simulink model "SMIB_pss"  (Simulink 8.7)
settings: Solver=ode3  StartTime=0.0  StopTime=10  FixedStep=1e-2  MaxStep=1e-2  RelTol=1e-5
values from neighbouring files (symbols this model uses):
  D = 0.0    (= 0)    [initDyn.m]
  delta0 = angle(v(2)+(Rs+1j*Xq)*IG0)    [initDyn.m]
  Efd0 = Epq0+(Xd-Xpd)*Id0    [initDyn.m]
  Epd0 = (Xq-Xpq)*Iq0    [initDyn.m]
  Epq0 = Vq0+Rs*Iq0+Xpd*Id0    [initDyn.m]
  event = [0 1 1.1 10 ... (first row only)    [initDyn.m]
  faulut_3ph = [ ... (first row only)    [initDyn.m]
  fYred = Yred    [initDyn.m]
  KA = ExData(:,1)    [initDyn.m]
  Kpss = KG*T1*T3/(T2*T4)    [initSSA.m]    (also in pss_test.m)
  M = 2*H/ws    [initDyn.m]
  small_d = [ ... (first row only)    [initDyn.m]
  T1 = x(2)    [initSSA.m]    (also in pss_test.m)
  T2 = x(3)    [initSSA.m]    (also in pss_test.m)
  T3 = x(4)    [initSSA.m]    (also in pss_test.m)
  T4 = x(5)    [initSSA.m]    (also in pss_test.m)
  TA = ExData(:,2)    [initDyn.m]
  Tpd0 = GenData(:,6)    [initDyn.m]
  Tpq0 = GenData(:,7)    [initDyn.m]
  Tw = 10    [initSSA.m]    (also in pss_test.m)
  Vinf = V0(1)    [initDyn.m]
  Vref1 = V0(2)+Efd0/KA    [initDyn.m]
  ws = 377    [initDyn.m]
  XXdpd = [Xd-Xpd]    [initDyn.m]
  XXpdq = [Xpq-Xpd]    [initDyn.m]
  XXqpq = [Xq-Xpq]    [initDyn.m]
  Yred = YN    [initDyn.m]
  Zdq = [Rsm -Xpqm;Xpdm Rsm]    [initDyn.m]
libraries: powerlib_extras x3
settings Model: Creator=hbeiran  LastModifiedBy=EBUKA
settings SolverCC: AlgebraicLoopSolver=LineSearch
settings DataIOCC: LimitDataPoints=off  SignalLoggingSaveFormat=ModelDataLogs
settings OptimizationCC: ExpressionDepthLimit=2147483647
settings DebuggingCC: AlgebraicLoopMsg=none  SolverPrmCheckMsg=warning  FcnCallInpInsideContextMsg=UseLocalSettings  StateNameClashWarn=warning
settings SFSimCC: SimParseCustomCode=off
settings GRTTargetCC: CombineOutputUpdateFcns=off  GRTInterface=on

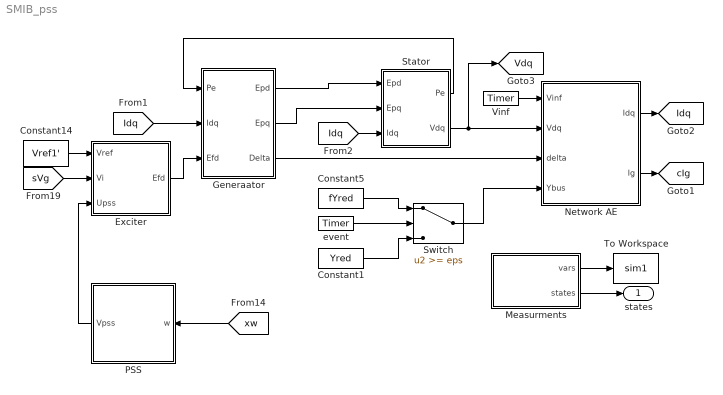
== system SMIB_pss ==
  Constant1 : Constant  Value=Yred  VectorParams1D=off
  Constant14 : Constant  Value=Vref1'  VectorParams1D=off
  Constant5 : Constant  Value=fYred  VectorParams1D=off
  Exciter : Subsystem
  Generaator : Subsystem
  Measurments : Subsystem
  Network AE : MATLAB Function  TreatAsAtomicUnit=on
  PSS : Subsystem
  Stator : Subsystem
  Switch : Switch  Threshold=eps
  To Workspace : ToWorkspace  VariableName=sim1  SaveFormat=Structure With Time  SampleTime=-1
  Vinf : powerlib_extras/Control  Blocks/Timer  t=faulut_3ph(1,:)  e=faulut_3ph(2,:)*Vinf
  event : powerlib_extras/Control  Blocks/Timer  t=event(1,:)  e=event(2,:)
  states : Outport
  tag scope: Idq=global, Vdq=global, cIg=global
  wires:
  Exciter/1(Efd) -> Generaator/3(Efd)
  Constant14/1 -> Exciter/1(Vref)
  [Idq] -> Generaator/2(Idq)
  Network AE/1(Idq) -> [Idq]
  event/1 -> Switch/2
  Constant5/1 -> Switch/1
  Constant1/1 -> Switch/3
  Switch/1 -> Network AE/4(Ybus)
  Measurments/1(vars) -> To Workspace/1
  Measurments/2(states) -> states/1
  Network AE/2(Ig) -> [cIg]
  Stator/2(Vdq) -> [Vdq], Network AE/2(Vdq)
  [Idq] -> Stator/3(Idq)
  Generaator/1(Epd) -> Stator/1(Epd)
  Generaator/2(Epq) -> Stator/2(Epq)
  Stator/1(Pe) -> Generaator/1(Pe)
  [sVg] -> Exciter/2(Vi)
  Vinf/1 -> Network AE/1(Vinf)
  Generaator/3(Delta) -> Network AE/3(delta)
  [xw] -> PSS/1(w)
  PSS/1(Vpss) -> Exciter/3(Upss)

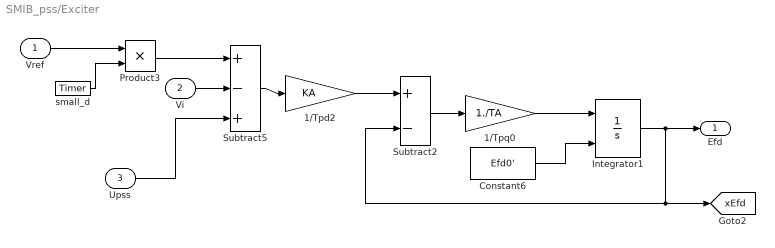
== system SMIB_pss/Exciter ==
  Vref : Inport
  Vi : Inport  Port=2
  Upss : Inport  Port=3
  1/Tpd2 : Gain  Gain=KA
  1/Tpq0 : Gain  Gain=1./TA
  Constant6 : Constant  Value=Efd0'  VectorParams1D=off
  Integrator1 : Integrator  InitialConditionSource=external
  Product3 : Product  RndMeth=Zero
  Subtract2 : Sum  Inputs=+-
  Subtract5 : Sum  Inputs=+-+
  small_d : powerlib_extras/Control  Blocks/Timer  t=small_d(1,:)  e=small_d(2,:)
  Efd : Outport
  tag scope: xEfd=global
  wires:
  Constant6/1 -> Integrator1/2
  Subtract2/1 -> 1/Tpq0/1
  1/Tpq0/1 -> Integrator1/1
  Integrator1/1 -> Efd/1, Subtract2/2, [xEfd]
  Vi/1 -> Subtract5/2
  Subtract5/1 -> 1/Tpd2/1
  1/Tpd2/1 -> Subtract2/1
  small_d/1 -> Product3/2
  Product3/1 -> Subtract5/1
  Vref/1 -> Product3/1
  Upss/1 -> Subtract5/3

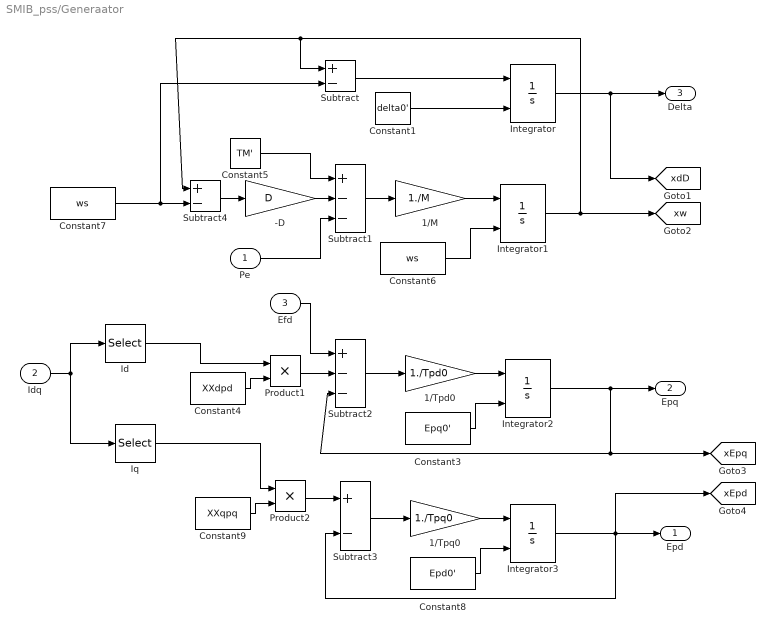
== system SMIB_pss/Generaator ==
  Pe : Inport
  Idq : Inport  Port=2
  Efd : Inport  Port=3
  -D : Gain  Gain=D
  1/M : Gain  Gain=1./M
  1/Tpd0 : Gain  Gain=1./Tpd0
  1/Tpq0 : Gain  Gain=1./Tpq0
  Constant1 : Constant  Value=delta0'  VectorParams1D=off
  Constant3 : Constant  Value=Epq0'  VectorParams1D=off
  Constant4 : Constant  Value=XXdpd  VectorParams1D=off
  Constant5 : Constant  Value=TM'  VectorParams1D=off
  Constant6 : Constant  Value=ws  VectorParams1D=off
  Constant7 : Constant  Value=ws  VectorParams1D=off
  Constant8 : Constant  Value=Epd0'  VectorParams1D=off
  Constant9 : Constant  Value=XXqpq  VectorParams1D=off
  Id : Selector  InputPortWidth=2  IndexOptions=Index vector (dialog)  Indices=[1]  OutputSizes=1
  Integrator{,1..3} (4 alike) : Integrator  InitialConditionSource=external
  Iq : Selector  InputPortWidth=2  IndexOptions=Index vector (dialog)  Indices=[2]  OutputSizes=1
  Product1 : Product  RndMeth=Zero
  Product2 : Product  RndMeth=Zero
  Subtract : Sum  Inputs=+-
  Subtract1 : Sum  Inputs=+--
  Subtract2 : Sum  Inputs=+--
  Subtract3 : Sum  Inputs=+-
  Subtract4 : Sum  Inputs=+-
  Epd : Outport
  Epq : Outport  Port=2
  Delta : Outport  Port=3
  tag scope: xEpd=global, xEpq=global, xdD=global, xw=global
  wires:
  Subtract/1 -> Integrator/1
  Constant5/1 -> Subtract1/1
  Subtract1/1 -> 1/M/1
  1/M/1 -> Integrator1/1
  Constant6/1 -> Integrator1/2
  -D/1 -> Subtract1/2
  Constant3/1 -> Integrator2/2
  Subtract2/1 -> 1/Tpd0/1
  Integrator2/1 -> Epq/1, Subtract2/3, [xEpq]
  Product1/1 -> Subtract2/2
  Constant4/1 -> Product1/2
  1/Tpd0/1 -> Integrator2/1
  Constant8/1 -> Integrator3/2
  Subtract3/1 -> 1/Tpq0/1
  Integrator3/1 -> Epd/1, [xEpd], Subtract3/2
  Constant9/1 -> Product2/2
  1/Tpq0/1 -> Integrator3/1
  Product2/1 -> Subtract3/1
  Efd/1 -> Subtract2/1
  Integrator1/1 -> Subtract/1, Subtract4/1, [xw]
  Id/1 -> Product1/1
  Idq/1 -> Id/1, Iq/1
  Iq/1 -> Product2/1
  Pe/1 -> Subtract1/3
  Integrator/1 -> Delta/1, [xdD]
  Subtract4/1 -> -D/1
  Constant7/1 -> Subtract4/2, Subtract/2
  Constant1/1 -> Integrator/2

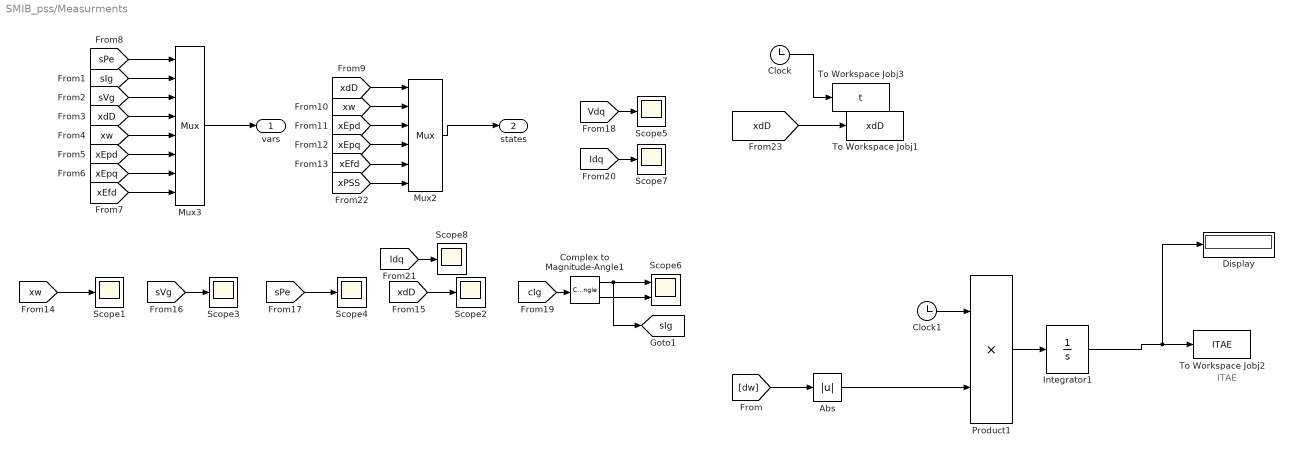
== system SMIB_pss/Measurments ==
  note: ITAE
  Abs : Abs
  Clock : Clock
  Clock1 : Clock
  Complex to Magnitude-Angle1 : ComplexToMagnitudeAngle
  Display : Display
  Integrator1 : Integrator
  Mux2 : Mux  Inputs=6
  Mux3 : Mux  Inputs=8
  Product1 : Product
  Scope{1..5,7..8} (7 alike) : Scope
  Scope6 : Scope  NumInputPorts=2
  To Workspace Jobj1 : ToWorkspace  VariableName=xdD  SampleTime=-1
  To Workspace Jobj2 : ToWorkspace  VariableName=ITAE  SampleTime=-1
  To Workspace Jobj3 : ToWorkspace  VariableName=t  SampleTime=-1
  vars : Outport
  states : Outport  Port=2
  tag scope: sIg=global
  wires:
  Mux3/1 -> vars/1
  [sPe] -> Mux3/1
  [sIg] -> Mux3/2
  [sVg] -> Mux3/3
  [xdD] -> Mux3/4
  [xw] -> Mux3/5
  [xEpd] -> Mux3/6
  [xEpq] -> Mux3/7
  [xEfd] -> Mux3/8
  [xw] -> Mux2/2
  [xEpd] -> Mux2/3
  [xEpq] -> Mux2/4
  [xEfd] -> Mux2/5
  [xdD] -> Mux2/1
  Mux2/1 -> states/1
  [xw] -> Scope1/1
  [xdD] -> Scope2/1
  [sVg] -> Scope3/1
  [sPe] -> Scope4/1
  Complex to Magnitude-Angle1/1 -> Scope6/1, [sIg]
  Complex to Magnitude-Angle1/2 -> Scope6/2
  [cIg] -> Complex to Magnitude-Angle1/1
  [Vdq] -> Scope5/1
  [Idq] -> Scope7/1
  [Idq] -> Scope8/1
  [xPSS] -> Mux2/6
  Clock/1 -> To Workspace Jobj3/1
  [xdD] -> To Workspace Jobj1/1
  Abs/1 -> Product1/2
  [dw] -> Abs/1
  Integrator1/1 -> Display/1, To Workspace Jobj2/1
  Clock1/1 -> Product1/1
  Product1/1 -> Integrator1/1

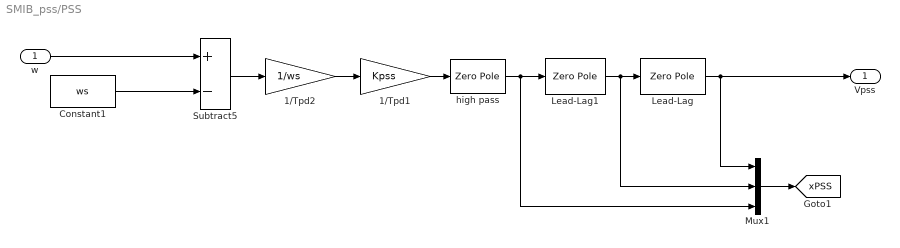
== system SMIB_pss/PSS ==
  w : Inport
  1/Tpd1 : Gain  Gain=Kpss
  1/Tpd2 : Gain  Gain=1/ws
  Constant1 : Constant  Value=ws  VectorParams1D=off
  Lead-Lag : ZeroPole  Zeros=[-1/T3]  Poles=[-1/T4]
  Lead-Lag1 : ZeroPole  Zeros=[-1/T1]  Poles=[-1/T2]
  Mux1 : Mux  Inputs=3
  Subtract5 : Sum  Inputs=+-
  high pass : ZeroPole  Zeros=[0]  Poles=[-1/Tw]
  Vpss : Outport
  tag scope: xPSS=global
  wires:
  Subtract5/1 -> 1/Tpd2/1
  1/Tpd1/1 -> high pass/1
  high pass/1 -> Lead-Lag1/1, Mux1/3
  Lead-Lag1/1 -> Lead-Lag/1, Mux1/2
  Mux1/1 -> [xPSS]
  1/Tpd2/1 -> 1/Tpd1/1
  Lead-Lag/1 -> Vpss/1, Mux1/1
  w/1 -> Subtract5/1
  Constant1/1 -> Subtract5/2

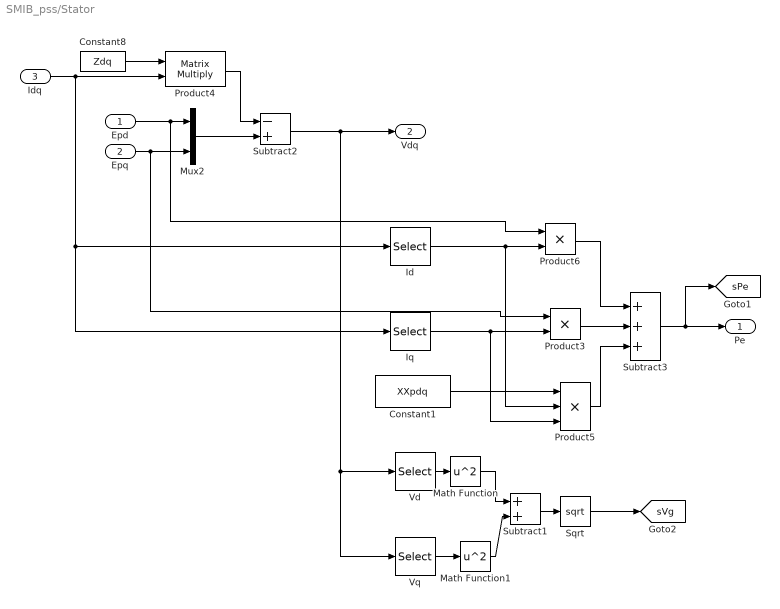
== system SMIB_pss/Stator ==
  Epd : Inport
  Epq : Inport  Port=2
  Idq : Inport  Port=3
  Constant1 : Constant  Value=XXpdq  VectorParams1D=off
  Constant8 : Constant  Value=Zdq  VectorParams1D=off
  Id : Selector  InputPortWidth=2  IndexOptions=Index vector (dialog)  Indices=[1]  OutputSizes=1
  Iq : Selector  InputPortWidth=2  IndexOptions=Index vector (dialog)  Indices=[2]  OutputSizes=1
  Math Function : Math  Operator=square  SaturateOnIntegerOverflow=on
  Math Function1 : Math  Operator=square  SaturateOnIntegerOverflow=on
  Mux2 : Mux  Inputs=2
  Product3 : Product  RndMeth=Zero
  Product4 : Product  Multiplication=Matrix(*)  RndMeth=Zero
  Product5 : Product  Inputs=3  RndMeth=Zero
  Product6 : Product  RndMeth=Zero
  Sqrt : Sqrt  SaturateOnIntegerOverflow=on
  Subtract1 : Sum
  Subtract2 : Sum  Inputs=-+
  Subtract3 : Sum  Inputs=+++
  Vd : Selector  InputPortWidth=2  IndexOptions=Index vector (dialog)  Indices=[1]  OutputSizes=1
  Vq : Selector  InputPortWidth=2  IndexOptions=Index vector (dialog)  Indices=[2]  OutputSizes=1
  Pe : Outport
  Vdq : Outport  Port=2
  tag scope: sPe=global, sVg=global
  wires:
  Constant8/1 -> Product4/1
  Epd/1 -> Mux2/1, Product6/1
  Epq/1 -> Product3/1, Mux2/2
  Iq/1 -> Product5/3, Product3/2
  Product6/1 -> Subtract3/1
  Product3/1 -> Subtract3/2
  Product5/1 -> Subtract3/3
  Constant1/1 -> Product5/1
  Subtract3/1 -> Pe/1, [sPe]
  Id/1 -> Product6/2, Product5/2
  Vd/1 -> Math Function/1
  Vq/1 -> Math Function1/1
  Math Function/1 -> Subtract1/1
  Math Function1/1 -> Subtract1/2
  Subtract1/1 -> Sqrt/1
  Sqrt/1 -> [sVg]
  Mux2/1 -> Subtract2/2
  Idq/1 -> Product4/2, Id/1, Iq/1
  Product4/1 -> Subtract2/1
  Subtract2/1 -> Vdq/1, Vq/1, Vd/1

== matlab function Network AE ==
  data: Vinf input double; Vdq input double; Idq output double; delta input double; Ig output double; Ybus input double
function [Idq, Ig] = fcn(Vinf, Vdq,delta,Ybus)
%#codegen
% global_var

% Idq

Tm = diag(exp(1j*(delta-pi/2)));
iTm = diag(exp(-1j*(delta-pi/2)));
% iTm = inv(Tm);
% Tm=eye(3);
Vg = Tm*(Vdq(1,1)+1j*Vdq(2,1));
% VLoad=VL(4:9,1);
Vbus=[Vinf;Vg];


I = Ybus*Vbus;
Ig=I(2,1);
Id=real(iTm*Ig);
Iq=imag(iTm*Ig);

Idq=[Id;Iq];
